simulink model "BuckyWagon_01"  (Simulink 7.5)
settings: Solver=FixedStepDiscrete  StartTime=0.0  StopTime=10.0  RelTol=1e-3
PreLoadFcn:
  | try, eval([bdroot '_setup']); catch, eval('model_setup', ''); end
InitFcn:
  | try, eval([bdroot '_setup']); catch, eval('model_setup', ''); end
undefined symbols (not defined in the file or in its folder): ECU565, High, Low, miniviewSetup, motohawk_build_version, motohawk_get_faults, motohawk_setup_toolchains, motohawk_trunc_name, motohawk_vardec_config_group, motohawk_vardec_path, tc, True
libraries: MotoHawk_lib x392, simulink x29, miniview_lib x10, motohawk_control_primitives_lib x9, motohawk_engine_lib x8, MotoHawk_VDOGauge_lib x8, motohawk_annotations_lib x2
(part 1 of 7)
Description:
  | ESled_08
CloseFcn:
  | try, eval([bdroot '_close']); catch, eval('model_close', ''); end
settings Model: MotoHawkBuildVersion=127  MotoHawkBuildStats=struct('TotalFLASH',{281540},'TotalEEPROM',{370},'TotalRAM',{18696},'AppFLASH',{71914},'AppEEPROM',{196},'AppRAM',{2166},'HeapRAM',{4096},'BuildSuccessCount',{130},'BuildErrorCount',{25},'OSRAM',{4754},'StackRAM',{7680},'FgndTimeStackSize',{3072},'FgndAngleStackSize',{0},'BgndStackSize',{2048},'IdleStackSize',{1024},'InterruptStackSize',{1536},'RTWBlockIOSize',{852},'RTWDWorkSize',{364},'RTWPrevZCSize',{0},'VolatileSize',{272},'NonVolatileSize',{196},'ConstantSize',{2208})  MotoHawkModelSavedName=BuckyWagon_01  MotoHawkModelGUID=3c32a120-d49a-4164-87-fe-ac-4b-55-ed-6f  MotoHawkModelOpenTime=2011 10 26 20 37 29.492  MotoHawkModelElapsedTime=-73544380.967  MotoHawkBuildInfo=struct('model_name',{'BuckyWagon_01'},'motohawk_version',{'2011a_sp0.184'},'motohawk_component_version',{'0.0.7'},'matlab_version',{'7.10.0'},'build_version',{'126'},'module_type',{'ECU565-128'},'layout_type',{'DEV'},'processor_family',{'PPC'},'processor_type',{'MPC565'},'toolchain_vendor',{'gcc-powerpc-eabi'},'toolchain_version',{'4.4.0'},'component',{0},'archive_file',{'PCM128.a'},'enable_build',{1},'fptype',{0},'flash_size',{1048576},'ee_size',{8192},'ram_size',{36864},'decram_size',{4096},'module_memory_def',{'MPC565_ModMemoryDef_Dev'},'eri_table0_rev',{9},'max_eri_table_size',{65535},'use_debug_vardecs',{1},'use_info_vardecs',{1},'fgnd_base_period_ms',{5},'bgnd_base_period_ms',{50},'root_build_dir',{'c:\motohawk\buckyWagon_01'},'build_dir',{'c:\motohawk\buckyWagon_01\BuckyWagon_01_Build'},'dll_name',{'BuckyWago_126'},'srz_name',{'BuckyWagon_01_126'},'fgnd_stack_size',{3072},'fgnd_angle_stack_size',{0},'bgnd_stack_size',{2048},'idle_stack_size',{1024},'irq_stack_size',{1536},'heap_size',{4096},'heap_margin',{409},'install_dll_dir',{'C:\ECUFiles\TDBDLL\'},'install_srz_dir',{'C:\ECUFiles\Programs'},'app_int_stack_size',{1024},'shutdown_stack_size',{1024},'mingw_dir',{'C:\PROGRA~2\Woodward\DEVELO~1\TOOLCH~1\GCC\win32-pe\4_4_0\'},'motohawk_dir',{'C:\PROGRA~2\Woodward\MCS\MotoHawk\2011A_~1.184'},'toolchain_dir',{'C:\Program Files (x86)\Woodward\DevelopmentTools\Toolchains\GCC\powerpc-eabi\4_4_0\'},'matlab_root',{'C:\MATLAB32'},'model_guid',{'3c32a120-d49a-4164-87-fe-ac-4b-55-ed-6f'},'build_guid',{'45c17ad0-7bc0-4506-bb-79-b7-2b-8f-43-7d'},'token_guid',{'7FCFF04D78B2574B8AB65D9942217FA2'})  MotoHawkBuildGUID=45c17ad0-7bc0-4506-bb-79-b7-2b-8f-43-7d  Creator=Danny  LastModifiedBy=Ethan
settings OptimizationCC: InlineParams=on  InitFltsAndDblsToZero=on  OptimizeModelRefInitCode=on  LifeSpan=1
settings DebuggingCC: SolverPrmCheckMsg=none  InheritedTsInSrcMsg=none  TasksWithSamePriorityMsg=none  StrictBusMsg=Warning
settings HardwareCC: ProdEndianess=BigEndian  ProdHWDeviceType=Specified
settings SFSimCC: SimCustomHeaderCode=|
  | #include <string.h>
  | #define charPtr(p) ((char *)p)
settings RTWCC: SystemTargetFile=motohawk_ert_rtw.tlc  TLCOptions="-aCustomNonFinites=\"motohawk_genrtnonfinite.tlc\""  MakeCommand=motohawk_make_rtw  TemplateMakefile=motohawk_ert_rtw.tmf  Description=MotoHawk(tm) Rapid Prototyping  ProcessScript=motohawk_ert_rtw_make_rtw_hook
settings CodeAppCC: IgnoreCustomStorageClasses=off  MaxIdLength=100  CustomSymbolStrField=$H$N$M
settings STFCustomTargetCC: ModelReferenceCompliant=off  CombineOutputUpdateFcns=on  ERTCustomFileBanners=on  SupportContinuousTime=off  SupportNonInlinedSFcns=off  SystemTargetFile=motohawk_ert_rtw.tlc
settings ERTTargetCC: MultiwordLength=2048  ModelReferenceCompliant=off  ParMdlRefBuildCompliant=off  CompOptLevelCompliant=off  ERTFirstTimeCompliant=off  ModelStepFunctionPrototypeControlCompliant=off  CPPClassGenCompliant=off  ERTCustomFileTemplate=example_file_process.tlc  ConvertIfToSwitch=off

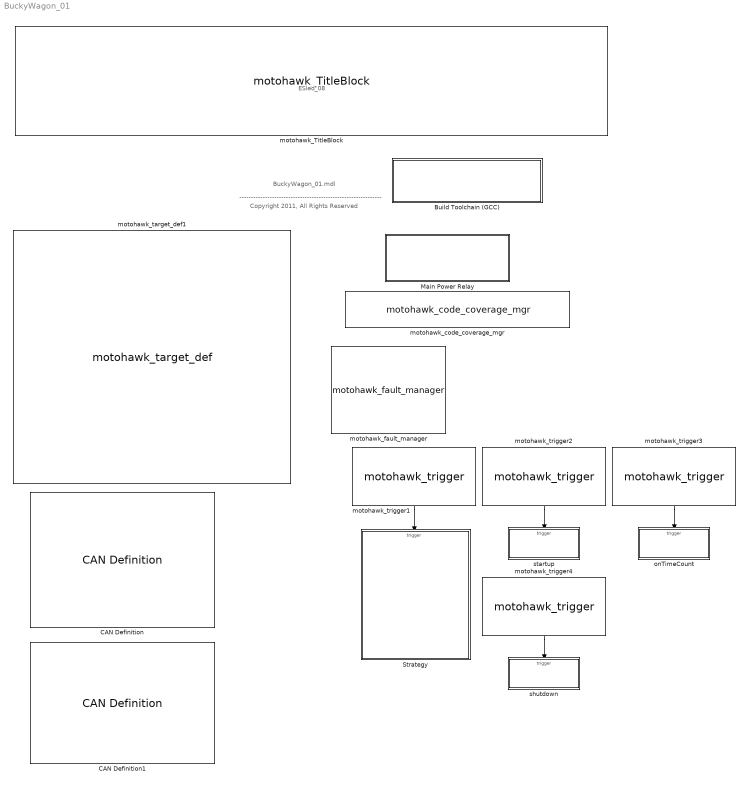
== system BuckyWagon_01 ==
  note: ESled_08
  note: BuckyWagon_01.mdl
  note: -------------------------------------------------------------
  note: Copyright 2011, All Rights Reserved
  Build Toolchain (GCC) : Subsystem
      mask Display:
      | patch([0 0 1 1], [0 1 1 0], [220/255 220/255 220/255]);
      | patch([0 0 1 1], [0 0.075 0.075 0], [230/255 0/255 0/255]);
      | patch([0 0 1 1], [0.025 0.05 0.05 0.025], [150/255 0/255 0/255]);
      | patch([0 0 1 1], [0 0.025 0.025 0], [0/255 0/255 0/255]);
      | 
      | disp(['Build'])
  CAN Definition : MotoHawk_lib/CAN Blocks/CAN Definition  Priority=-100  nam=['CAN_' num2str(1)]  text_resource=CAN1  code_resource=NONE  val_resource=-1  target=ECU565-128  bus=-2  btime=250 kbaud  pre=1  prop=0  pseg1=0  pseg2=0  resyn=0  tx_queue_size=16  rx_queue_size=16  use_protocol=on  city_id=hex2dec('B')  access_level=4  mototune_group='System | System Config | Communication Config'
  CAN Definition1 : MotoHawk_lib/CAN Blocks/CAN Definition  Priority=-100  nam=['CAN_' num2str(2)]  text_resource=CAN2  code_resource=NONE  val_resource=-1  target=ECU565-128  bus=-2  btime=500 kbaud  pre=1  prop=0  pseg1=0  pseg2=0  resyn=0  tx_queue_size=16  rx_queue_size=16  use_protocol=off  city_id=hex2dec('B')  access_level=4  mototune_group='System | System Config | Communication Config'
  Main Power Relay : Subsystem  AncestorBlock=MotoHawk_lib/Extra Development Blocks/Main Power Relay  mask(MotoHawk Main Power Relay Control){on_delay_count=2, off_delay_count=10, ecup_threshold=100, group='System | Main Power Relay'}
      mask prompts: on_delay_count "On Delay Count"; off_delay_count "Off Delay Count"; ecup_threshold "ECUP High Threshold (ADC Counts)"; group "MotoTune Group"
      mask help:
      | This block provides basic control of the main power relay, by following the ECUP voltage input pin.
      |
      | Regardless of where the block is placed in a design, the strategy will execute every 50ms with background priority.
      |
      | Note that this block is simply composed of other primitive MotoHawk blocks and may be used as a starting point for a more complicated strategy.
      |
      | On Delay:  Once the ECU power goes high, after this period, the Main Power Relay will be turned on.
      | Off Delay:  Once the ECU power goes low, after this period, the Main Power Relay will be turned off.
      |
      | Note that one tick before MPRD is turned off, non-volatile variables will be stored, and the Shutdown event will be posted.  It is not necessary to use the Shutdown event.
      |
      | ---------------------------------------------------------------------
      |
      |
      | Copyright 2010 Woodward.  All Rights Reserved.
      mask init:
      | block = gcb;
      | 
      | motohawk_main_power_relay_initmask;
      mask Help: eval('motohawk_block_help(get_param(gcb,''MaskType''))');
      mask Display:
      | patch([0 0 1 1], [0 1 1 0], [220/255 220/255 220/255]);
      | patch([0 0 1 1], [0 0.075 0.075 0], [230/255 0/255 0/255]);
      | patch([0 0 1 1], [0.025 0.05 0.05 0.025], [150/255 0/255 0/255]);
      | patch([0 0 1 1], [0 0.025 0.025 0], [0/255 0/255 0/255]);
      | 
      | disp(['Main Power Relay' on_delay_lbl off_delay_lbl]);
  Strategy : Subsystem  TreatAsAtomicUnit=on
      settings: RTWSystemCode=Function  RTWFcnNameOpts=Use subsystem name  RTWFileNameOpts=Use function name
  motohawk_TitleBlock : motohawk_annotations_lib/motohawk_TitleBlock  BlockType_='Mototron_Title_Block'  ttl="[  strrep(get_param(bdroot, 'Description') , '_', '\\_')  '\\newline\\rm'  'Top-level root of model:  '   strrep(bdroot, '_', '\\_') '.mdl'  ]"  copyright="'THE INFORMATION CONTAINED IN THIS\\newlineDRAWING IS THE SOLE PROPERTY OF\\newlineMOTOTRON.  ANY REPRODUCTION IN\\newline PART OR AS A WHOLE WITHOUT THE\\newlineWRITTEN PERMISSION OF MOTOTRON\\newline IS PROHIBITED.\\fontsize{16}\\rm\\copyright\\rm\\fontsize{10} 2005'"  address='\fontsize{22}\it\fontname{Arial Black}MotoTron Corporation \fontname{Arial}\fontsize{10}\newline505 Marion Road, Oshkosh, WI, 54901\newlinewww.mototron.com (734) 822-7700'  image_file='mh.jpg'  pretty_print=on  edit_text=|  edit_as=5
      | [	
      | 
      | 
      | 	
      | 
      | 
      | strrep(get_param(bdroot, 'Description') , '_', '\_')  '\newline\rm'	
      | 
      | 
      | 	
      | 
      | 
      | 'Top-level root of model:  '   strrep(bdroot, '_', '\_') '.mdl'	
      | 
      | 
      | 	
      | 
      | 
      | ]
  motohawk_code_coverage_mgr : MotoHawk_lib/Extra Development Blocks/motohawk_code_coverage_mgr  codegen=Always Generate Code Coverage Code  group='System | Code Coverage'
  motohawk_fault_manager : MotoHawk_lib/Fault Management Blocks/motohawk_fault_manager  storage=FLASH  read_level=1  write_level=1  clear_level=1  xytype=uint16  mototune_group='Faults'
  motohawk_target_def1 : MotoHawk_lib/motohawk_target_def  Priority=-65535  target=ECU565-128  layout=DEV  fptype=single (32 bits)  fgnd_stack_size=3*1024  fgnd_angle_stack_size=0  bgnd_stack_size=2*1024  idle_stack_size=1024  irq_stack_size=1536  app_int_stack_size=1024  shutdown_stack_size=1024  heap_size=4*1024  show_margins=off  fgnd_stack_margin=(3*1024) * 0.1  fgnd_angle_stack_margin=0  bgnd_stack_margin=(2*1024) * 0.1  idle_stack_margin=(1024) * 0.1  irq_stack_margin=(1536) * 0.1  app_int_stack_margin=(1024) * 0.1  shutdown_stack_margin=(1024) * 0.1  heap_margin=(4*1024) * 0.1  comp_name=bdroot  comp_img='KVASER_CAN_USB.jpg'  comp_security=No Encryption  comp_build_pass='mhbuild'  comp_sim_pass='mhsim'  comp_multi=off  show_filenames=off  dll_name=motohawk_trunc_name(bdroot, ['_' motohawk_build_version], 13)  srz_name=motohawk_trunc_name(bdroot, ['_' motohawk_build_version], 50)  build_dir='.'  comp_dir='.'
  motohawk_trigger1 : MotoHawk_lib/Trigger Blocks/motohawk_trigger  Tag=Trigger  trigger=FGND_RTI_PERIODIC  function_name=Trigger_FGND_RTI_PERIODIC_9090p0107  priority_order=0  inherited=off  run_disabled=off  override_app_monitor=off  target=ECU565_128
  motohawk_trigger2 : MotoHawk_lib/Trigger Blocks/motohawk_trigger  Tag=Trigger  trigger=STARTUP_EVENT  function_name=Trigger_STARTUP_EVENT_9091p0016  priority_order=0  inherited=off  run_disabled=off  override_app_monitor=off  target=ECU565_128
  motohawk_trigger3 : MotoHawk_lib/Trigger Blocks/motohawk_trigger  Tag=Trigger  trigger=BGND_BASEx20_PERIODIC  function_name=Trigger_BGND_BASEx20_PERIODIC_9092p0017  priority_order=0  inherited=off  run_disabled=off  override_app_monitor=off  target=ECU565_128
  motohawk_trigger4 : MotoHawk_lib/Trigger Blocks/motohawk_trigger  Tag=Trigger  Priority=0  trigger=SHUTDOWN_EVENT  function_name=Trigger_SHUTDOWN_EVENT_9093p0017  priority_order=0  inherited=off  run_disabled=off  override_app_monitor=off  target=ECU565_128
  onTimeCount : Subsystem  TreatAsAtomicUnit=on
  shutdown : Subsystem  TreatAsAtomicUnit=on
  startup : Subsystem  TreatAsAtomicUnit=on
  wires:
  motohawk_trigger1/1 -> Strategy/Trigger
  motohawk_trigger2/1 -> startup/Trigger
  motohawk_trigger3/1 -> onTimeCount/Trigger
  motohawk_trigger4/1 -> shutdown/Trigger

== system BuckyWagon_01/Build Toolchain (GCC) ==
  note: MotoHawk
  note: ---------------------------------------------------------------------
      | Copyright 2010 Woodward.  All Rights Reserved.
  note: Build Blocks
  Tool Chain Definition : S-Function  InitFcn=motohawk_setup_toolchains(gcb, 'init');  FunctionName=motohawk_sfun_toolchain_def  Parameters=char({tc,''})  EnableBusSupport=off  mask(MotoHawk Tool Chain Definition){nam='MyToolChain', toolchain=gcc-powerpc-eabi 4.4.0, buildtemplate=GreenHills 3.6, toolchaindir='C:\GHS\ppc421\', target=ECU565-128}
      mask prompts: nam "Name"; toolchain "Tool Chain"; buildtemplate "Build Template"; toolchaindir "Tool Chain Install Directory"; target "Target (hidden)"
      mask help:
      | This block chooses the tool chain for MotoHawk to use when CTRL+B is pressed.
      |
      | The "Name" is a user-specified name given to the tool chain.  It has no bearing on the tool chain chosen, it is for documentation purposes.
      |
      | The "Tool Chain" drop down list contains the tool chains that are available for this target.
      |
      | A "Custom" toolchain allows the user to choose an alternate directory with a supported build template.
      |
      | The "Build template" will force MotoHawk to generate build scripts and files for the specified tool chain.  Note that a custom tool chain must be compatible with a supported tool chain, otherwise the build will not succeed.
      |
      | ---------------------------------------------------------------------
      |
      |
      | Copyright 2010 Woodward.  All Rights Reserved.
      mask init:
      | block = gcb;
      | 
      | motohawk_sfun_toolchain_def_initmask;
      settings: OpenFcn=|
      | motohawk_setup_toolchains(gcb, 'open');
      | open_system(gcb, 'mask');
      mask Help: eval('motohawk_block_help(get_param(gcb,''MaskType''))');
      mask StyleString: edit,popup((None)|(Custom)|GreenHills 3.6|GreenHills 4.2.1|gcc-powerpc-eabi 4.4.0),popup(GreenHills 3.6|GreenHills 4.2.1|gcc-powerpc-eabi 4.4.0),edit,edit
      mask CallbackString: |motohawk_sfun_toolchain_def_visible(gcb)|||
      mask Display:
      | patch([0 0 1 1], [0 1 1 0], [220/255 220/255 220/255]);
      | 
      | patch([0 0 1 1], [0 0.075 0.075 0], [230/255 0/255 0/255]);
      | patch([0 0 1 1], [0.025 0.05 0.05 0.025], [150/255 0/255 0/255]);
      | 
      | patch([0 0 1 1], [0 0.025 0.025 0], [0/255 0/255 0/255]);
      | 
      | 
      | text(0.1, 0.9, lbl, 'texmode', 'on', 'HorizontalAlignment', 'Left', 'VerticalAlignment', 'Top');

== system BuckyWagon_01/Main Power Relay ==
  note: Always execute Main Power Relay control in the background.
  note: The saving and restoring of non-volatile variables
      | must be called from a background priority task.
  Background : Subsystem
  motohawk_trigger : MotoHawk_lib/Trigger Blocks/motohawk_trigger  Tag=Trigger  Priority=255  trigger=BGND_BASE_PERIODIC  function_name=Trigger_BGND_BASE_PERIODIC_190p0018  priority_order=255  inherited=on  run_disabled=on  override_app_monitor=off  target=ECU565_128
  wires:
  motohawk_trigger/1 -> Background/Trigger

== system BuckyWagon_01/Strategy ==
  function : TriggerPort  TriggerType=function-call
  Actuators : Subsystem
  Control Strategy : Subsystem
  Gauges : Subsystem
  MiniViewDisplay : Subsystem
      settings: RTWSystemCode=Function  RTWFcnNameOpts=Use subsystem name  RTWFileNameOpts=Use function name
  Sensors : Subsystem
  motohawk_trigger : MotoHawk_lib/Trigger Blocks/motohawk_trigger  Tag=Trigger  trigger=FGND_RTI_PERIODIC  function_name=Trigger_FGND_RTI_PERIODIC_9072p0017  priority_order=200  inherited=on  run_disabled=off  override_app_monitor=off  target=ECU565_128
  motohawk_trigger1 : MotoHawk_lib/Trigger Blocks/motohawk_trigger  Tag=Trigger  trigger=FGND_20XRTI_PERIODIC  function_name=Trigger_FGND_20XRTI_PERIODIC_9073p002  priority_order=200  inherited=on  run_disabled=off  override_app_monitor=off  target=ECU565_128
  wires:
  Sensors/1(Sensors) -> Control Strategy/1(Inputs), Gauges/1(Inputs), MiniViewDisplay/1(Inputs)  "Physical"
  Control Strategy/1(Outputs) -> Actuators/1(Outputs), Gauges/2(Outputs), MiniViewDisplay/2(Outputs)  "Hybrid"
  motohawk_trigger/1 -> MiniViewDisplay/Trigger
  motohawk_trigger1/1 -> Gauges/Trigger

== system BuckyWagon_01/onTimeCount ==
  function : TriggerPort  TriggerType=function-call
  Constant : Constant  OutDataTypeMode=uint32  OutDataType=sfix(16)  OutScaling=2^0  OutDataTypeStr=uint32
  Sum : Sum  Inputs=++|  OutDataType=sfix(16)  OutScaling=2^0
  motohawk_data_def : MotoHawk_lib/Data Storage Blocks/motohawk_data_def  nam='totalOnTime'  container_nam=''  data=0  typ=uint32  struct_nam='MyStruct'  storage=NonVolatile  outputRef=on  use_vardec=on  window=Display  read_level=1  write_level=1  ovr_cals=on  view_as=Number  enum_struct={'Disabled', 'Enabled'}  vector_style=Wide Row  use_help_units=off  help=''  units=''  use_header_enum=off  row_header_enum=''  col_header_enum=''  use_min_max=off  min_val=-inf  max_val=inf  use_precision=off  precision=''  gain=1  offset=0  exp=1  use_mototune_group=off  mototune_group=motohawk_vardec_path(gcb)  eval_name=MyData  data_stores=motohawk_sfun_data_def_data_stores  struct_instances=motohawk_sfun_data_def_struct_instances  vardecs=motohawk_sfun_data_def_vardecs
  motohawk_data_read : MotoHawk_lib/Data Storage Blocks/motohawk_data_read  source=Input Reference Signal  structure=Scalar  operation=Read scalar from location by index  sz_vec=4  sz_row=2  sz_col=3  typ=uint32  nam='MyData'  checkNull=on  struct_inst_name=''  struct_nam='MyStruct'
  motohawk_data_write : MotoHawk_lib/Data Storage Blocks/motohawk_data_write  source=Input Reference Signal  structure=Scalar  operation=Write entire data structure at once  sz_vec=9  sz_row=2  sz_col=9  typ=uint32  nam='MyData'  checkNull=on  write_read_only=off  struct_inst_name=''  struct_name='MyStruct'
  wires:
  Constant/1 -> Sum/1
  Sum/1 -> motohawk_data_write/1
  motohawk_data_read/1 -> Sum/2
  motohawk_data_def/1 -> motohawk_data_write/2, motohawk_data_read/1

== system BuckyWagon_01/shutdown ==
  function : TriggerPort  TriggerType=function-call
  VDO Gauge Reset : MotoHawk_VDOGauge_lib/VDO Gauge Reset  nam='GaugeChain'

== system BuckyWagon_01/startup ==
  function : TriggerPort  TriggerType=function-call
  Constant : Constant  OutDataTypeMode=uint32  OutDataType=sfix(16)  OutScaling=2^0  OutDataTypeStr=uint32
  Sum : Sum  Inputs=++|  OutDataType=sfix(16)  OutScaling=2^0
  VDO Gauge Reset : MotoHawk_VDOGauge_lib/VDO Gauge Reset  nam='GaugeChain'
  motohawk_data_def : MotoHawk_lib/Data Storage Blocks/motohawk_data_def  nam='startupCount'  container_nam=''  data=0  typ=uint32  struct_nam='MyStruct'  storage=NonVolatile  outputRef=on  use_vardec=on  window=Display  read_level=1  write_level=1  ovr_cals=on  view_as=Number  enum_struct={'Disabled', 'Enabled'}  vector_style=Wide Row  use_help_units=off  help=''  units=''  use_header_enum=off  row_header_enum=''  col_header_enum=''  use_min_max=off  min_val=-inf  max_val=inf  use_precision=off  precision=''  gain=1  offset=0  exp=1  use_mototune_group=off  mototune_group=motohawk_vardec_path(gcb)  eval_name=MyData  data_stores=motohawk_sfun_data_def_data_stores  struct_instances=motohawk_sfun_data_def_struct_instances  vardecs=motohawk_sfun_data_def_vardecs
  motohawk_data_read : MotoHawk_lib/Data Storage Blocks/motohawk_data_read  source=Input Reference Signal  structure=Scalar  operation=Read scalar from location by index  sz_vec=4  sz_row=2  sz_col=3  typ=uint32  nam='MyData'  checkNull=on  struct_inst_name=''  struct_nam='MyStruct'
  motohawk_data_write : MotoHawk_lib/Data Storage Blocks/motohawk_data_write  source=Input Reference Signal  structure=Scalar  operation=Write entire data structure at once  sz_vec=9  sz_row=2  sz_col=9  typ=uint32  nam='MyData'  checkNull=on  write_read_only=off  struct_inst_name=''  struct_name='MyStruct'
  wires:
  motohawk_data_def/1 -> motohawk_data_read/1, motohawk_data_write/2
  motohawk_data_read/1 -> Sum/2
  Sum/1 -> motohawk_data_write/1
  Constant/1 -> Sum/1

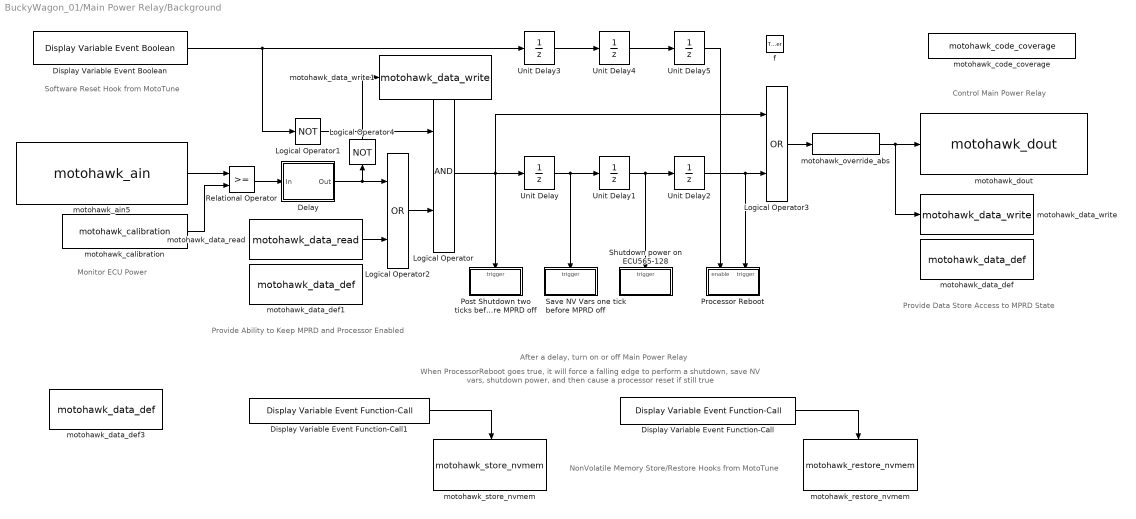
== system BuckyWagon_01/Main Power Relay/Background ==
  note: Monitor ECU Power
  note: After a delay, turn on or off Main Power Relay
  note: When ProcessorReboot goes true, it will force a falling edge to perform a shutdown, save NV vars, shutdown power, and then cause a processor reset if still true
  note: Software Reset
      | Hook from MotoTune
  note: NonVolatile Memory Store/Restore
      | Hooks from MotoTune
  note: Control Main Power Relay
  note: Provide Data Store
      | Access to MPRD State
  note: Provide Ability to Keep
      | MPRD and Processor Enabled
  f : TriggerPort  TriggerType=function-call  ZeroCross=off
  Delay : Subsystem
  Display Variable Event Boolean : MotoHawk_lib/Extra Development Blocks/Display Variable Event Boolean  SystemSampleTime=-1  nam='ProcessorReboot'  level=1  enum_str={'Run', 'Reboot'}  help_str='Reboots the processor when set.'  group=group
  Display Variable Event Function-Call : MotoHawk_lib/Extra Development Blocks/Display Variable Event Function-Call  SystemSampleTime=-1  nam='RestoreNVFactoryDefaults'  level=1  enum_str={'Run', 'Restore To Defaults'}  help_str='Restores NonVolatile Memory to Factory Defaults'  group='System | NonVolatile Storage'
  Display Variable Event Function-Call1 : MotoHawk_lib/Extra Development Blocks/Display Variable Event Function-Call  SystemSampleTime=-1  nam='StoreNV'  level=1  enum_str={'Run', 'Store To EEPROM'}  help_str='Stores RAM-Shadowed memory to serial EEPROM'  group='System | NonVolatile Storage'
  Logical Operator : Logic  OutDataTypeMode=boolean  OutDataTypeStr=boolean
  Logical Operator1 : Logic  Operator=NOT  OutDataTypeMode=boolean  OutDataTypeStr=boolean
  Logical Operator2 : Logic  Operator=OR  OutDataTypeMode=boolean  OutDataTypeStr=boolean
  Logical Operator3 : Logic  Operator=OR  OutDataTypeMode=boolean  OutDataTypeStr=boolean
  Logical Operator4 : Logic  Operator=NOT  OutDataTypeMode=boolean  OutDataTypeStr=boolean
  Post Shutdown two ticks before MPRD off : Subsystem
  Processor Reboot : Subsystem  TreatAsAtomicUnit=on
  Relational Operator : RelationalOperator  LogicOutDataTypeMode=boolean  OutDataTypeStr=boolean  ZeroCross=off  InputSameDT=on
  Save NV Vars one tick before MPRD off : Subsystem
  Shutdown power on ECU565-128 : Subsystem
  Unit Delay{,1..5} (6 alike) : UnitDelay  SampleTime=-1
  motohawk_ain5 : MotoHawk_lib/Analog I//O Blocks/motohawk_ain  res_name=[]  text_resource=ECUP  code_resource=NONE  val_resource=-1  target=ECU565-128  resource_enum_str=(None)=-1,ECUP=53,DRVP=54,XDRP=55,AN1M=56,AN2M=57,AN3M=58,AN4M=59,AN5M=60,AN6M=61,AN7M=62,AN8M=63,AN9M=64,AN10M=65,AN11M=66,AN12M=67,AN13M=68,AN14M=69,AN15M=70,AN16M=71,AN17M=72,AN18M=73,AN19M=74,AN20M=75,AN21M=76,AN22M=77,AN23M=78,AN24M=79,AN25M=80,AN26M=81,AN27M=82,AN28M=83,AN29M=84,AN30M=85,AN31M=86,AN32M=87,AN33M=88,AN34M=89,O2A=90,O2B=91,XDRP_B=92,REF_14V=143  altref=5V Reference  typ=uint16  num_adc_bits=10  use_stat=off  use_vardec=off  nam='AIN'  read_level=1  write_level=1  group='System | I/O Pins | Inputs Config'
  motohawk_calibration : MotoHawk_lib/Calibration & Probing Blocks/motohawk_calibration  nam='ECUP_Threshold'  val=ecup_threshold  storage=Calibration  show_more=on  name_source=Use Parameter  data_type=uint16  read_level=1  write_level=1  ovr_cals=on  view_as=Number  enum_struct={'Disabled', 'Enabled'}  vector_style=Wide Row  use_help_units=off  help='ADC voltage threshold above which ECU is considered powered'  units='ADC_counts'  use_header_enum=off  row_header_enum={}  col_header_enum={}  use_min_max=on  min_val=0  max_val=1023  use_precision=off  precision=''  gain=1  offset=0  exp=1  use_mototune_group=on  mototune_group=motohawk_vardec_config_group(group)
  motohawk_code_coverage : MotoHawk_lib/Extra Development Blocks/motohawk_code_coverage
  motohawk_data_def : MotoHawk_lib/Data Storage Blocks/motohawk_data_def  nam='MPRD'  container_nam=''  data=false  typ=Inherit from 'Initial Value'  struct_nam='MyStruct'  storage=Volatile  outputRef=off  use_vardec=on  window=Display  read_level=1  write_level=(Read Only)  ovr_cals=on  view_as=Enumeration  enum_struct={'Disabled', 'Enabled'}  vector_style=Wide Row  use_help_units=off  help='Indicates whether the main power relay is active'  units=''  use_header_enum=off  row_header_enum={}  col_header_enum={}  use_min_max=off  min_val=0  max_val=1  use_precision=off  precision=''  gain=1  offset=0  exp=1  use_mototune_group=on  mototune_group=group  eval_name=MPRD  data_stores=motohawk_sfun_data_def_data_stores  struct_instances=motohawk_sfun_data_def_struct_instances  vardecs=motohawk_sfun_data_def_vardecs
  motohawk_data_def1 : MotoHawk_lib/Data Storage Blocks/motohawk_data_def  nam='MPRD_KeepAlive'  container_nam=''  data=false  typ=Inherit from 'Initial Value'  struct_nam='MyStruct'  storage=Volatile  outputRef=off  use_vardec=on  window=Display  read_level=1  write_level=1  ovr_cals=on  view_as=Enumeration  enum_struct={'Disable on low ECUP', 'Keep alive'}  vector_style=Wide Row  use_help_units=on  help='When enabled, keeps the MPRD output on and keeps the processor alive'  units=''  use_header_enum=off  row_header_enum={}  col_header_enum={}  use_min_max=off  min_val=0  max_val=1  use_precision=off  precision=''  gain=1  offset=0  exp=1  use_mototune_group=on  mototune_group=group  eval_name=MPRD_KeepAlive  data_stores=motohawk_sfun_data_def_data_stores  struct_instances=motohawk_sfun_data_def_struct_instances  vardecs=motohawk_sfun_data_def_vardecs
  motohawk_data_def3 : MotoHawk_lib/Data Storage Blocks/motohawk_data_def  nam='Shutdown_Req'  container_nam=''  data=false  typ=boolean  struct_nam='MyStruct'  storage=Volatile  outputRef=off  use_vardec=on  window=Display  read_level=1  write_level=1  ovr_cals=on  view_as=Number  enum_struct={'Disable on low ECUP', 'Keep alive'}  vector_style=Wide Row  use_help_units=on  help=''  units=''  use_header_enum=off  row_header_enum={}  col_header_enum={}  use_min_max=off  min_val=0  max_val=1  use_precision=off  precision=''  gain=1  offset=0  exp=1  use_mototune_group=on  mototune_group=group  eval_name=MPRD_KeepAlive  data_stores=motohawk_sfun_data_def_data_stores  struct_instances=motohawk_sfun_data_def_struct_instances  vardecs=motohawk_sfun_data_def_vardecs
  motohawk_data_read : MotoHawk_lib/Data Storage Blocks/motohawk_data_read  source=Lookup By Name  structure=Scalar  operation=Read scalar from location by index  sz_vec=4  sz_row=2  sz_col=3  typ=boolean  nam='MPRD_KeepAlive'  checkNull=on  struct_inst_name='Struct1'  struct_nam='MyStruct'
  motohawk_data_write : MotoHawk_lib/Data Storage Blocks/motohawk_data_write  source=Lookup By Name  structure=Scalar  operation=Write entire data structure at once  sz_vec=-1  sz_row=3  sz_col=2  typ=boolean  nam='MPRD'  checkNull=off  write_read_only=off  struct_inst_name='Struct1'  struct_name='MyStruct'
  motohawk_data_write1 : MotoHawk_lib/Data Storage Blocks/motohawk_data_write  source=Lookup By Name  structure=Scalar  operation=Write entire data structure at once  sz_vec=-1  sz_row=3  sz_col=2  typ=boolean  nam='Shutdown_Req'  checkNull=off  write_read_only=off  struct_inst_name='Struct1'  struct_name='MyStruct'
  motohawk_dout : MotoHawk_lib/Digital I//O Blocks/motohawk_dout  resource_name=[]  text_resource=MPRD  target=ECU565-128  use_diag=off  use_vardec=off  nam='DOUT'  read_level=1  write_level=1  group='System | I/O Pins | Outputs Config'
  motohawk_override_abs : MotoHawk_lib/Calibration & Probing Blocks/motohawk_override_abs  SystemSampleTime=-1  parent_name='MPRD'  parent_val=0  show_more=on  name_source=Use Parameter  parent_read_level=1  parent_override_level=1  view_as=Enumeration  enum_struct={'Off', 'On'}  use_help_units=off  parent_help='Directly Override Main Power Relay'  parent_units='boolean'  use_min_max=on  parent_min=0  parent_max=1  use_precision=off  parent_precision=''  parent_gain=1  parent_offset=0  parent_exp=1  use_mototune_group=on  parent_group=group
  motohawk_restore_nvmem : MotoHawk_lib/Data Storage Blocks/motohawk_restore_nvmem  SystemSampleTime=-1
  motohawk_store_nvmem : MotoHawk_lib/Data Storage Blocks/motohawk_store_nvmem  SystemSampleTime=-1
  wires:
  motohawk_override_abs/1 -> motohawk_data_write/1, motohawk_dout/1
  motohawk_ain5/1 -> Relational Operator/1
  motohawk_calibration/1 -> Relational Operator/2
  Relational Operator/1 -> Delay/1(In)
  Unit Delay/1 -> Unit Delay1/1, Save NV Vars one tick before MPRD off/Trigger
  Unit Delay1/1 -> Shutdown power on ECU565-128/Trigger, Unit Delay2/1
  Display Variable Event Boolean/1 -> Logical Operator1/1, Unit Delay3/1
  Logical Operator/1 -> Post Shutdown two ticks before MPRD off/Trigger, Unit Delay/1, Logical Operator3/1
  Logical Operator1/1 -> Logical Operator/1
  Unit Delay2/1 -> Processor Reboot/Trigger, Logical Operator3/2
  Display Variable Event Function-Call/1 -> motohawk_restore_nvmem/Trigger
  Display Variable Event Function-Call1/1 -> motohawk_store_nvmem/Trigger
  Unit Delay3/1 -> Unit Delay4/1
  Unit Delay4/1 -> Unit Delay5/1
  Unit Delay5/1 -> Processor Reboot/Enable
  Logical Operator2/1 -> Logical Operator/2
  Delay/1(Out) -> Logical Operator2/1, Logical Operator4/1
  motohawk_data_read/1 -> Logical Operator2/2
  Logical Operator3/1 -> motohawk_override_abs/1
  Logical Operator4/1 -> motohawk_data_write1/1

== system BuckyWagon_01/Strategy/Actuators ==
  Outputs : Inport  OutDataType=sfix(16)  OutScaling=2^0
  A123 Battery Controller : Subsystem  TreatAsAtomicUnit=on
  Brusa Charger : Subsystem  AncestorBlock=motohawk_annotations_lib/Display Image File  mask(Display Image File){image_file='NLG5.jpg'}
      mask prompts: image_file "Image File"
      mask help:
      | Enter an image file on the current MATLAB path to display on this block.
      |
      | Double-clicking this block opens the contents of the subsystem.  Right-click and select 'Mask parameters...' to select a new image file.
      |
      | To use just the mask of this block in a model, but supply your own contents, break the link to the library.
      mask init:
      | try,
      | 	img = imread(image_file);
      | 	motohawk_block_image(gcb, image_file);
      | catch,
      | 	img = imread('image_not_found.jpg');
      | end
      settings: OpenFcn=open_system(gcb,'force');  MoveFcn=motohawk_block_image(gcb, motohawk_get_param_ws(gcb, 'image_file'));
      mask Display: image(img);
  Bus Selector1 : BusSelector  OutputSignals=Phoenix Enable,motor_torque
  Bus Selector2 : BusSelector  OutputSignals=InReverse,WaterPumpDuty
  Bus Selector3 : BusSelector  OutputSignals=Contactor Command
  Bus Selector4 : BusSelector  OutputSignals=EHPAS Enable
  Bus Selector5 : BusSelector  OutputSignals=NLG5
  Bus Selector6 : BusSelector  OutputSignals=EHPAS Enable
  Bus Selector7 : BusSelector  OutputSignals=OilPumpDutyCycle
  Cruise Control Indicator : Subsystem
  DC/DC Converter Controller : Subsystem  TreatAsAtomicUnit=on
  Discrete Actuator Characterization1 : motohawk_engine_lib/Discrete Actuator Characterization  SystemSampleTime=-1  prefix='RevOut_'  nam='ReverseOut'  units='bool'  parent_group='Actuators | Reverse'  polarity=High-True
  EHPAS Power Steering Pump Controller : Subsystem  TreatAsAtomicUnit=on
  Logical Operator3 : Logic  Operator=OR  IconShape=distinctive  AllPortsSameDT=off  OutDataTypeMode=boolean  OutDataTypeStr=boolean
  PWM Characterization1 : motohawk_engine_lib/PWM Characterization  SystemSampleTime=-1  nam='WaterPumpOut'  prefix='WtrPmpOut_'  units='%'  parent_group='Actuators | WaterPump'
  PWM Characterization2 : motohawk_engine_lib/PWM Characterization  SystemSampleTime=-1  nam='OilPumpOut'  prefix='OilPumpOut_'  units='%'  parent_group='Actuators | OilPump'
      link override motohawk_calibration2: val=-100
  Phoenix Drive Controller : Subsystem  TreatAsAtomicUnit=on
  ReverseInd : Subsystem
  motohawk_dout1 : MotoHawk_lib/Digital I//O Blocks/motohawk_dout  resource_name=[]  text_resource=(None)  target=ECU565-128  use_diag=off  use_vardec=on  nam='ReverseOut_Pin'  read_level=1  write_level=1  group='System | I/O Pins | Outputs Config'
  motohawk_pwm1 : MotoHawk_lib/Analog I//O Blocks/motohawk_pwm  res_name=[]  text_resource=(None)  code_resource=NONE  val_resource=-1  target=ECU565-128  resource_enum_str=(None)=-1,H1=1,H2=10,FINJ1=12,FINJ2=13,FINJ3=14,FINJ4=15,FINJ5=16,FINJ6=17,FINJ7=18,FINJ8=19,FINJ9=20,FINJ10=21,FINJ11=22,FINJ12=23,TACH=24,LSD1=25,LSD2=26,LSD3=27,LSD4=28,LSD5=29,LSD6=30,LSD7=31,LSD8=32,LSD9=33,LSD10=34,EST 1=36,EST 2=37,EST 3=38,EST 4=39,EST 5=40,EST 6=41,EST 7=42,EST 8=43,EST 9=44,EST 10=45,EST 11=46,EST 12=47,EST 13=48,EST 14=49,EST 15=50,EST 16=51,H3=107  freq_mode=-1  min_freq=2  use_max_freq=off  max_freq=42949672.96  use_enable=off  use_brake=off  output_current=off  output_fault_status=off  use_child=off  use_vardec=on  nam='WaterPump_Pin'  read_level=1  write_level=1  group='System | I/O Pins | Outputs Config'
  motohawk_pwm2 : MotoHawk_lib/Analog I//O Blocks/motohawk_pwm  res_name=[]  text_resource=(None)  code_resource=NONE  val_resource=-1  target=ECU565-128  resource_enum_str=(None)=-1,H1=1,H2=10,FINJ1=12,FINJ2=13,FINJ3=14,FINJ4=15,FINJ5=16,FINJ6=17,FINJ7=18,FINJ8=19,FINJ9=20,FINJ10=21,FINJ11=22,FINJ12=23,TACH=24,LSD1=25,LSD2=26,LSD3=27,LSD4=28,LSD5=29,LSD6=30,LSD7=31,LSD8=32,LSD9=33,LSD10=34,EST 1=36,EST 2=37,EST 3=38,EST 4=39,EST 5=40,EST 6=41,EST 7=42,EST 8=43,EST 9=44,EST 10=45,EST 11=46,EST 12=47,EST 13=48,EST 14=49,EST 15=50,EST 16=51,H3=107  freq_mode=-1  min_freq=2  use_max_freq=off  max_freq=42949672.96  use_enable=off  use_brake=off  output_current=off  output_fault_status=off  use_child=off  use_vardec=on  nam='OilPump_Pin'  read_level=1  write_level=1  group='System | I/O Pins | Outputs Config'
  wires:
  Discrete Actuator Characterization1/1 -> motohawk_dout1/1
  Outputs/1 -> Bus Selector1/1, Bus Selector4/1, Bus Selector5/1, Bus Selector2/1, Bus Selector7/1, Bus Selector6/1, Bus Selector3/1
  PWM Characterization1/1 -> motohawk_pwm1/1
  PWM Characterization1/2 -> motohawk_pwm1/2
  Bus Selector2/2 -> PWM Characterization1/1  "<WaterPumpDuty>"
  Bus Selector2/1 -> ReverseInd/1(In)  "<InReverse>"
  Cruise Control Indicator/1(Out) -> Logical Operator3/1
  ReverseInd/1(Out) -> Logical Operator3/2
  Logical Operator3/1 -> Discrete Actuator Characterization1/1
  Bus Selector5/1 -> Brusa Charger/1(In1)  "<NLG5>"
  Bus Selector1/2 -> Phoenix Drive Controller/2(Torque Command)  "<motor_torque>"
  Bus Selector3/1 -> A123 Battery Controller/1(Contactor Command)  "<Contactor Command>"
  Bus Selector1/1 -> Phoenix Drive Controller/1(Drive Enable)  "<Phoenix Enable>"
  Bus Selector4/1 -> EHPAS Power Steering Pump Controller/1(Enable)  "<EHPAS Enable>"
  Bus Selector6/1 -> DC/DC Converter Controller/1(Enable)  "<EHPAS Enable>"
  PWM Characterization2/1 -> motohawk_pwm2/1
  PWM Characterization2/2 -> motohawk_pwm2/2
  Bus Selector7/1 -> PWM Characterization2/1  "<OilPumpDutyCycle>"

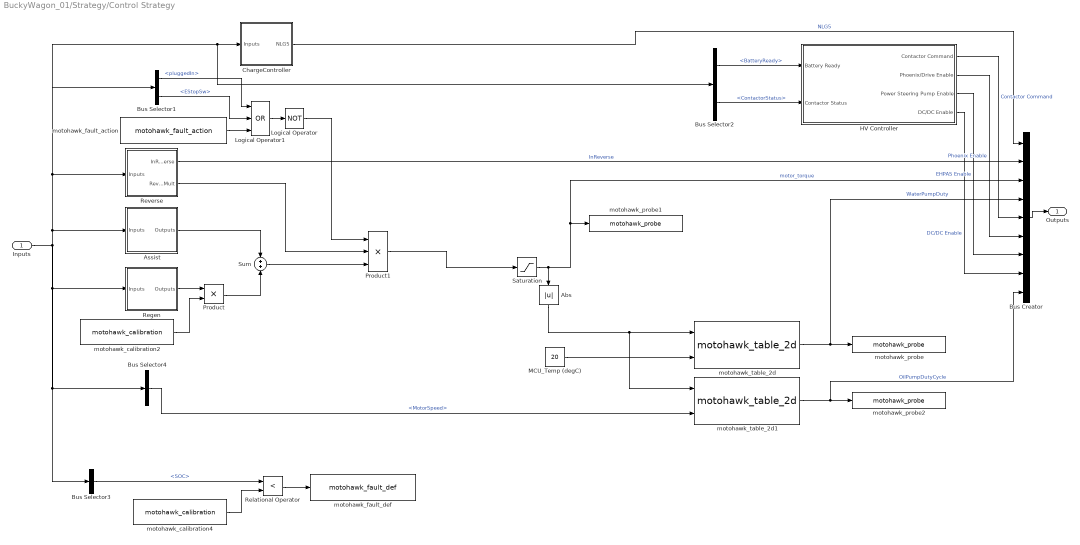
== system BuckyWagon_01/Strategy/Control Strategy ==
  Inputs : Inport  OutDataType=sfix(16)  OutScaling=2^0
  Abs : Abs
  Assist : Subsystem  TreatAsAtomicUnit=on
  Bus Creator : BusCreator  Inputs=9
  Bus Selector1 : BusSelector  OutputSignals=NLG5.pluggedIn,EStopSw
  Bus Selector2 : BusSelector  OutputSignals=BatteryReady,ContactorStatus
  Bus Selector3 : BusSelector  OutputSignals=SOC
  Bus Selector4 : BusSelector  OutputSignals=MotorSpeed
  ChargeController : Subsystem  TreatAsAtomicUnit=on
  HV Controller : Subsystem  TreatAsAtomicUnit=on
  Logical Operator : Logic  Operator=NOT  AllPortsSameDT=off  OutDataTypeMode=boolean  OutDataTypeStr=boolean
  Logical Operator1 : Logic  Operator=OR  Inputs=3  AllPortsSameDT=off  OutDataTypeMode=boolean  OutDataTypeStr=boolean
  MCU_Temp (degC) : Constant  Value=20  OutDataType=fixdt(1, 16)  OutScaling=2^0
  Product : Product  OutDataType=sfix(16)  OutScaling=2^0  RndMeth=Zero
  Product1 : Product  Inputs=3  OutDataType=sfix(16)  OutScaling=2^0  RndMeth=Zero
  Regen : Subsystem  TreatAsAtomicUnit=on
  Relational Operator : RelationalOperator  Operator=<  LogicOutDataTypeMode=boolean  OutDataTypeStr=boolean
  Reverse : Subsystem  TreatAsAtomicUnit=on
  Saturation : Saturate  UpperLimit=1  LowerLimit=-1
  Sum : Sum  OutDataType=sfix(16)  OutScaling=2^0
  motohawk_calibration2 : MotoHawk_lib/Calibration & Probing Blocks/motohawk_calibration  nam='Regen_Enable'  val=0  storage=Calibration  show_more=on  name_source=Use Parameter  data_type=Inherit from 'Default Value'  read_level=1  write_level=1  ovr_cals=on  view_as=Number  enum_struct={'Disabled', 'Enabled'}  vector_style=Wide Row  use_help_units=on  help='Enables Regen Braking'  units=''  use_header_enum=off  row_header_enum={}  col_header_enum={}  use_min_max=off  min_val=0  max_val=1  use_precision=on  precision='1.0'  gain=1  offset=0  exp=1  use_mototune_group=off  mototune_group=motohawk_vardec_path(gcb)
  motohawk_calibration4 : MotoHawk_lib/Calibration & Probing Blocks/motohawk_calibration  nam='SOC_Dead'  val=0.03  storage=Calibration  show_more=on  name_source=Use Parameter  data_type=Inherit from 'Default Value'  read_level=1  write_level=1  ovr_cals=on  view_as=Number  enum_struct={'Disabled', 'Enabled'}  vector_style=Wide Row  use_help_units=on  help='Below this SOC a Batt Dead fault will occur.'  units='%'  use_header_enum=off  row_header_enum={}  col_header_enum={}  use_min_max=on  min_val=0  max_val=1  use_precision=on  precision='1.3'  gain=1  offset=0  exp=1  use_mototune_group=off  mototune_group=motohawk_vardec_path(gcb)
  motohawk_fault_action : MotoHawk_lib/Fault Management Blocks/motohawk_fault_action  nam='DisableDrive'  output_status=on  eval_nam=DisableDrive
  motohawk_fault_def : MotoHawk_lib/Fault Management Blocks/motohawk_fault_def  nam='BattDead'  mode=Enabled  id=0  x=100  y=200  input_suspected=on  indeterminate=off  increment_xy=on  downsample_count=1  ovr_cals=on  ovr_actions=off  show_actions=off  action1_name=''  action1_cond=(None)  action2_name=''  action2_cond=(None)  action3_name=''  action3_cond=(None)  action4_name=''  action4_cond=(None)
  motohawk_probe : MotoHawk_lib/Calibration & Probing Blocks/motohawk_probe  nam='WaterPumpDuty'  show_more=off  name_source=Use Parameter  read_level=1  view_as=Number  enum_struct={'Disabled', 'Enabled'}  vector_style=Wide Row  use_help_units=off  help=''  units=''  use_header_enum=off  row_header_enum={}  col_header_enum={}  use_precision=off  precision=''  gain=1  offset=0  exp=1  use_mototune_group=off  mototune_group=motohawk_vardec_path(gcb)
  motohawk_probe1 : MotoHawk_lib/Calibration & Probing Blocks/motohawk_probe  nam='motor_Torque'  show_more=on  name_source=Use Parameter  read_level=1  view_as=Number  enum_struct={'Disabled', 'Enabled'}  vector_style=Wide Row  use_help_units=off  help=''  units=''  use_header_enum=off  row_header_enum={}  col_header_enum={}  use_precision=on  precision='1.3'  gain=1  offset=0  exp=1  use_mototune_group=off  mototune_group=motohawk_vardec_path(gcb)
  motohawk_probe2 : MotoHawk_lib/Calibration & Probing Blocks/motohawk_probe  nam='OilPumpDutyCycle'  show_more=off  name_source=Use Parameter  read_level=1  view_as=Number  enum_struct={'Disabled', 'Enabled'}  vector_style=Wide Row  use_help_units=off  help=''  units=''  use_header_enum=off  row_header_enum={}  col_header_enum={}  use_precision=off  precision=''  gain=1  offset=0  exp=1  use_mototune_group=off  mototune_group=motohawk_vardec_path(gcb)
  motohawk_table_2d : MotoHawk_lib/Lookup Tables/motohawk_table_2d  SystemSampleTime=-1  nam='WaterPumpDutyMap'  row_nam='MotorTorque'  col_nam='MCUTemp'  row_breakpoint_data=[0 0.1 0.2 0.3 0.4 0.5 0.6 0.7 0.8 0.9 1]  col_breakpoint_data=[0 10 20 30 40 50 60 70 80 90 100]  table_data=[1 1 1 1 1 1 1 1 1 1 1;1 1 1 1 1 1 1 1 1 1 1;1 1 1 1 1 1 1 1 1 1 1;1 1 1 1 1 1 1 1 1 1 1;1 1 1 1 1 1 1 1 1 1 1;1 1 1 1 1 1 1 1 1 1 1;1 1 1 1 1 1 1 1 1 1 1;1 1 1 1 1 1 1 1 1 1 1;1 1 1 1 1 1 1 1 1 1 1;1 1 1 1 1 1 1 1 1 1 1;1 1 1 1 1 1 1 1 1 1 1]  show_more=off  row_bp_data_type=Inherit from 'Row Breakpoint Data'  col_bp_data_type=Inherit from 'Column Breakpoint Data'  bp_storage=Constant  table_data_type=Inherit from 'Table Data'  storage=NonAdaptive  read_level=1  write_level=1  ovr_cals=on  use_help=off  help=''  row_bp_units=''  col_bp_units=''  table_units=''  use_min_max=off  row_bp_min_val=-inf  row_bp_max_val=inf  col_bp_min_val=-inf  col_bp_max_val=inf  min_val=-inf  max_val=inf  use_precision=off  use_row_breakpoint=off  rb_precision=''  rb_gain=1  rb_offset=0  rb_exp=1  use_col_breakpoint=off  cb_precision=''  cb_gain=1  cb_offset=0  cb_exp=1  use_table=off  t_precision=''  t_gain=1  t_offset=0  t_exp=1  use_links=off  row_input_name=''  col_input_name=''  output_name=''  use_mototune_group=off  mototune_group=motohawk_vardec_path(gcb)
  motohawk_table_2d1 : MotoHawk_lib/Lookup Tables/motohawk_table_2d  SystemSampleTime=-1  nam='OilPumpDuty'  row_nam='MotorTorqueX'  col_nam='MotorSpeedX'  row_breakpoint_data=[0 0.1 0.2 0.3 0.4 0.5 0.6 0.7 0.8 0.9 1]  col_breakpoint_data=[0 10 20 30 40 50 60 70 80 90 100]  table_data=[1 1 1 1 1 1 1 1 1 1 1;1 1 1 1 1 1 1 1 1 1 1;1 1 1 1 1 1 1 1 1 1 1;1 1 1 1 1 1 1 1 1 1 1;1 1 1 1 1 1 1 1 1 1 1;1 1 1 1 1 1 1 1 1 1 1;1 1 1 1 1 1 1 1 1 1 1;1 1 1 1 1 1 1 1 1 1 1;1 1 1 1 1 1 1 1 1 1 1;1 1 1 1 1 1 1 1 1 1 1;1 1 1 1 1 1 1 1 1 1 1]  show_more=off  row_bp_data_type=Inherit from 'Row Breakpoint Data'  col_bp_data_type=Inherit from 'Column Breakpoint Data'  bp_storage=Constant  table_data_type=Inherit from 'Table Data'  storage=NonAdaptive  read_level=1  write_level=1  ovr_cals=on  use_help=off  help=''  row_bp_units=''  col_bp_units=''  table_units=''  use_min_max=off  row_bp_min_val=-inf  row_bp_max_val=inf  col_bp_min_val=-inf  col_bp_max_val=inf  min_val=-inf  max_val=inf  use_precision=off  use_row_breakpoint=off  rb_precision=''  rb_gain=1  rb_offset=0  rb_exp=1  use_col_breakpoint=off  cb_precision=''  cb_gain=1  cb_offset=0  cb_exp=1  use_table=off  t_precision=''  t_gain=1  t_offset=0  t_exp=1  use_links=off  row_input_name=''  col_input_name=''  output_name=''  use_mototune_group=off  mototune_group=motohawk_vardec_path(gcb)
  Outputs : Outport  OutDataType=sfix(16)  OutScaling=2^0
  wires:
  Inputs/1 -> Assist/1(Inputs), Reverse/1(Inputs), Bus Selector1/1, Regen/1(Inputs), Bus Selector3/1, ChargeController/1(Inputs), Bus Selector2/1, Bus Selector4/1
  Saturation/1 -> motohawk_probe1/1, Bus Creator/3, Abs/1  "motor_torque"
  Regen/1(Outputs) -> Product/1
  motohawk_calibration2/1 -> Product/2
  Assist/1(Outputs) -> Sum/1
  Product/1 -> Sum/2
  Reverse/2(ReverseMult) -> Product1/2
  Product1/1 -> Saturation/1
  Sum/1 -> Product1/3
  Logical Operator/1 -> Product1/1
  Reverse/1(InReverse) -> Bus Creator/2  "InReverse"
  Bus Creator/1 -> Outputs/1
  Abs/1 -> motohawk_table_2d/1, motohawk_table_2d1/1
  MCU_Temp (degC)/1 -> motohawk_table_2d/2
  motohawk_table_2d/1 -> motohawk_probe/1, Bus Creator/4  "WaterPumpDuty"
  Bus Selector1/2 -> Logical Operator1/2  "<EStopSw>"
  motohawk_fault_action/1 -> Logical Operator1/3
  Logical Operator1/1 -> Logical Operator/1
  Bus Selector1/1 -> Logical Operator1/1  "<pluggedIn>"
  ChargeController/1(NLG5) -> Bus Creator/1  "NLG5"
  motohawk_calibration4/1 -> Relational Operator/2
  Relational Operator/1 -> motohawk_fault_def/1
  Bus Selector3/1 -> Relational Operator/1  "<SOC>"
  Bus Selector2/1 -> HV Controller/1(Battery Ready)  "<BatteryReady>"
  Bus Selector2/2 -> HV Controller/2(Contactor Status)  "<ContactorStatus>"
  HV Controller/1(Contactor Command) -> Bus Creator/5  "Contactor Command"
  HV Controller/2(Phoenix/Drive Enable) -> Bus Creator/6  "Phoenix Enable"
  HV Controller/3(Power Steering Pump Enable) -> Bus Creator/7  "EHPAS Enable"
  HV Controller/4(DC/DC Enable) -> Bus Creator/8  "DC/DC Enable"
  motohawk_table_2d1/1 -> motohawk_probe2/1, Bus Creator/9  "OilPumpDutyCycle"
  Bus Selector4/1 -> motohawk_table_2d1/2  "<MotorSpeed>"
